simulink model "RAKANSL"  (R2020a)
settings: Solver=VariableStepAuto  StartTime=0.0  StopTime=10.0  RelTol=1e-3
values from neighbouring files (symbols this model uses):
  Ct = 1    [RAKAN.m]
  Cw = 1    [RAKAN.m]
  Kt = 1    [RAKAN.m]
  Kw = 1    [RAKAN.m]
  mB = 1    [RAKAN.m]
  mu = 1    [RAKAN.m]
settings Model: Creator=crist  LastModifiedBy=crist

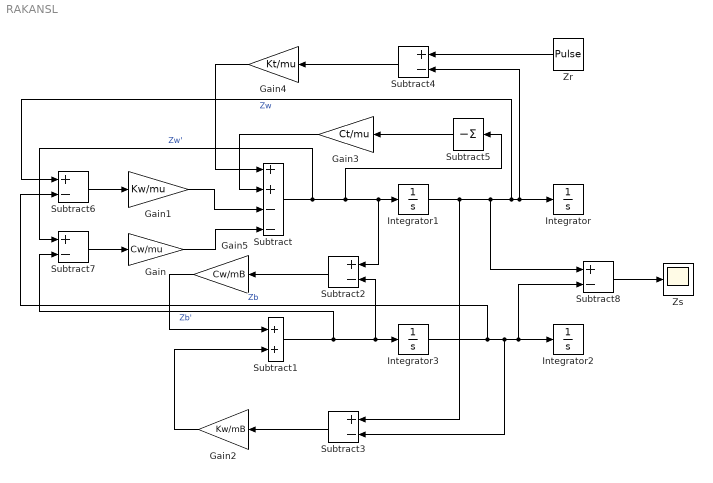
== system RAKANSL ==
  Gain : Gain  Gain=Cw/mu
  Gain1 : Gain  Gain=Kw/mu
  Gain2 : Gain  Gain=Kw/mB
  Gain3 : Gain  Gain=Ct/mu
  Gain4 : Gain  Gain=Kt/mu
  Gain5 : Gain  Gain=Cw/mB
  Integrator{,1..3} (4 alike) : Integrator
  Subtract : Sum  Inputs=++--
  Subtract1 : Sum
  Subtract{2..4,6..8} (6 alike) : Sum  Inputs=+-
  Subtract5 : Sum  Inputs=-
  Zr : DiscretePulseGenerator  PulseType=Time based  Period=10  PulseWidth=5
  Zs : Scope
  wires:
  Integrator1/1 -> Subtract3/1, Subtract8/1, Subtract6/1, Subtract4/2, Integrator/1  "Zw"
  Integrator3/1 -> Subtract6/2, Subtract3/2, Subtract8/2, Integrator2/1  "Zb"
  Subtract1/1 -> Subtract7/2, Subtract2/2, Integrator3/1  "Zb'"
  Subtract/1 -> Subtract7/1, Subtract5/1, Subtract2/1, Integrator1/1  "Zw'"
  Gain5/1 -> Subtract1/1
  Subtract2/1 -> Gain5/1
  Subtract3/1 -> Gain2/1
  Gain2/1 -> Subtract1/2
  Zr/1 -> Subtract4/1
  Subtract4/1 -> Gain4/1
  Gain4/1 -> Subtract/1
  Gain3/1 -> Subtract/2
  Subtract5/1 -> Gain3/1
  Gain1/1 -> Subtract/3
  Subtract6/1 -> Gain1/1
  Gain/1 -> Subtract/4
  Subtract7/1 -> Gain/1
  Subtract8/1 -> Zs/1
